simulink model "three_phase_Gen_SpeedControl"  (R2023b)
settings: Solver=VariableStepAuto  StartTime=0.0  StopTime=10.0  RelTol=1e-3
undefined symbols (not defined in the file): rated, Ts
libraries: mcbcontrolslib x2
settings Model: Creator=ela19kfs  LastModifiedBy=Legion

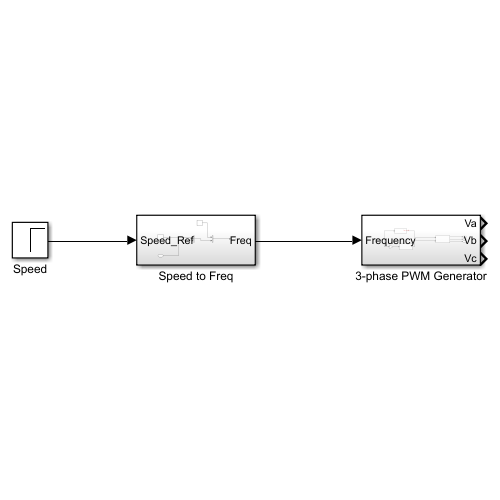
[thumbnail: Simulink's stored preview of the top-level diagram]
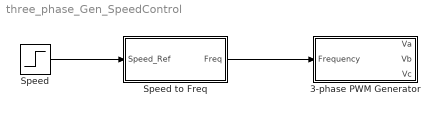
== system three_phase_Gen_SpeedControl ==
  3-phase PWM Generator : Subsystem
  Speed : Step  SampleTime=0
  Speed to Freq : Subsystem
  wires:
  Speed/1 -> Speed to Freq/1(Speed_Ref)
  Speed to Freq/1(Freq) -> 3-phase PWM Generator/1(Frequency)

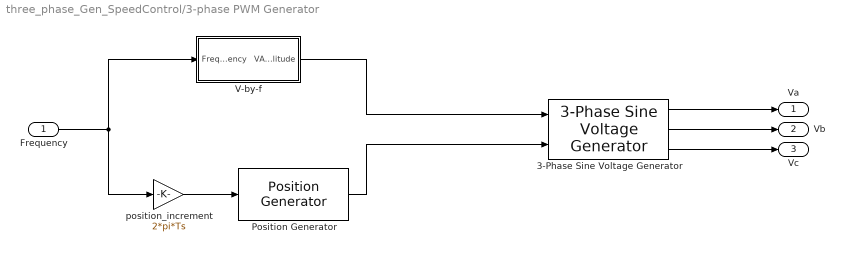
== system three_phase_Gen_SpeedControl/3-phase PWM Generator ==
  Frequency : Inport
  3-Phase Sine Voltage Generator : mcbcontrolslib/3-Phase Sine Voltage Generator  AngleInput=Radians  N_points=1024
  Position Generator : mcbcontrolslib/Position Generator  AngleOutput=Radians  ExternalReset=none  Offset=0
  V-by-f : Subsystem
  position_increment : Gain  Gain=2*pi*Ts  RndMeth=Simplest  OutDataTypeStr=Inherit: Same as input
  Va : Outport
  Vb : Outport  Port=2
  Vc : Outport  Port=3
  wires:
  V-by-f/1(VAmplitude) -> 3-Phase Sine Voltage Generator/1
  3-Phase Sine Voltage Generator/3 -> Vc/1
  ? -> ?
  position_increment/1 -> Position Generator/1
  3-Phase Sine Voltage Generator/1 -> Va/1
  3-Phase Sine Voltage Generator/2 -> Vb/1
  Frequency/1 -> V-by-f/1(Frequency), position_increment/1
  Position Generator/1 -> 3-Phase Sine Voltage Generator/2

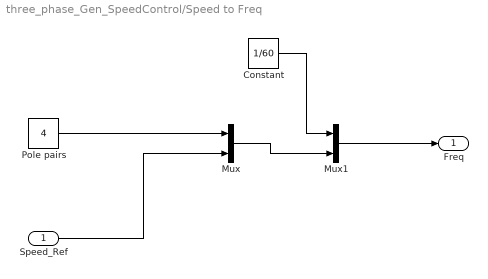
== system three_phase_Gen_SpeedControl/Speed to Freq ==
  Speed_Ref : Inport
  Constant : Constant  Value=1/60
  Mux : Mux  Inputs=2
      settings: DisplayOption=signals
  Mux1 : Mux  Inputs=2
  Pole pairs : Constant  Value=4
  Freq : Outport
  wires:
  Speed_Ref/1 -> Mux/2
  Pole pairs/1 -> Mux/1
  Constant/1 -> Mux1/1
  Mux/1 -> Mux1/2
  Mux1/1 -> Freq/1

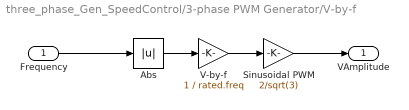
== system three_phase_Gen_SpeedControl/3-phase PWM Generator/V-by-f ==
  Frequency : Inport
  Abs : Abs  RndMeth=Simplest  SaturateOnIntegerOverflow=off
  Sinusoidal PWM : Gain  Gain=2/sqrt(3)  RndMeth=Simplest  OutDataTypeStr=Inherit: Same as input
  V-by-f : Gain  Gain=1 / rated.freq  RndMeth=Simplest  OutDataTypeStr=Inherit: Same as input
  VAmplitude : Outport
  wires:
  Abs/1 -> V-by-f/1
  V-by-f/1 -> Sinusoidal PWM/1
  Frequency/1 -> Abs/1
  Sinusoidal PWM/1 -> VAmplitude/1
